simulink model "sum_multi_test"  (Simulink 8.4)
settings: Solver=VariableStepDiscrete  StartTime=0.0  StopTime=10.0  RelTol=1e-3
settings Model: Creator=arnaud  LastModifiedBy=arnaud
settings DataIOCC: SaveFormat=Structure
settings DebuggingCC: StrictBusMsg=Warning

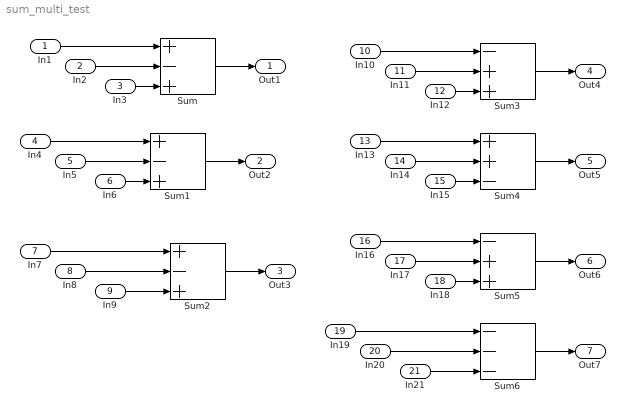
== system sum_multi_test ==
  In1 : Inport
  In2 : Inport  Port=2
  In3 : Inport  Port=3
  In4 : Inport  Port=4  PortDimensions=3
  In5 : Inport  Port=5  PortDimensions=3
  In6 : Inport  Port=6  PortDimensions=3
  In7 : Inport  Port=7  PortDimensions=[2 3]
  In8 : Inport  Port=8  PortDimensions=[2 3]
  In9 : Inport  Port=9  PortDimensions=[2 3]
  In10 : Inport  Port=10  PortDimensions=1
  In11 : Inport  Port=11  PortDimensions=3
  In12 : Inport  Port=12  PortDimensions=1
  In13 : Inport  Port=13  PortDimensions=3
  In14 : Inport  Port=14  PortDimensions=1
  In15 : Inport  Port=15  PortDimensions=3
  In16 : Inport  Port=16  PortDimensions=1
  In17 : Inport  Port=17  PortDimensions=[2 3]
  In18 : Inport  Port=18  PortDimensions=1
  In19 : Inport  Port=19  PortDimensions=[2 3]
  In20 : Inport  Port=20  PortDimensions=1
  In21 : Inport  Port=21  PortDimensions=[2 3]
  Sum : Sum  Inputs=+-+
  Sum1 : Sum  Inputs=+-+
  Sum2 : Sum  Inputs=+-+
  Sum3 : Sum  Inputs=-++
  Sum4 : Sum  Inputs=++-
  Sum5 : Sum  Inputs=-++
  Sum6 : Sum  Inputs=---
  Out1 : Outport
  Out2 : Outport  Port=2
  Out3 : Outport  Port=3
  Out4 : Outport  Port=4
  Out5 : Outport  Port=5
  Out6 : Outport  Port=6
  Out7 : Outport  Port=7
  wires:
  In1/1 -> Sum/1
  Sum/1 -> Out1/1
  In2/1 -> Sum/2
  In3/1 -> Sum/3
  In4/1 -> Sum1/1
  Sum1/1 -> Out2/1
  In5/1 -> Sum1/2
  In6/1 -> Sum1/3
  In7/1 -> Sum2/1
  Sum2/1 -> Out3/1
  In8/1 -> Sum2/2
  In9/1 -> Sum2/3
  In10/1 -> Sum3/1
  Sum3/1 -> Out4/1
  In11/1 -> Sum3/2
  In12/1 -> Sum3/3
  In13/1 -> Sum4/1
  Sum4/1 -> Out5/1
  In14/1 -> Sum4/2
  In15/1 -> Sum4/3
  In16/1 -> Sum5/1
  Sum5/1 -> Out6/1
  In17/1 -> Sum5/2
  In18/1 -> Sum5/3
  In19/1 -> Sum6/1
  Sum6/1 -> Out7/1
  In20/1 -> Sum6/2
  In21/1 -> Sum6/3
